simulink model "fir"  (R2019b)
settings: Solver=VariableStepAuto  StartTime=0.0  StopTime=inf  RelTol=1e-3
undefined symbols (not defined in the file): S, vsva2197, xcvc1902, xlfda_numerator
libraries: ModelComposer x2, xbsIndex_r4 x1, dspsrcs4 x1
settings Model: Creator=abehbood  LastModifiedBy=viswanad

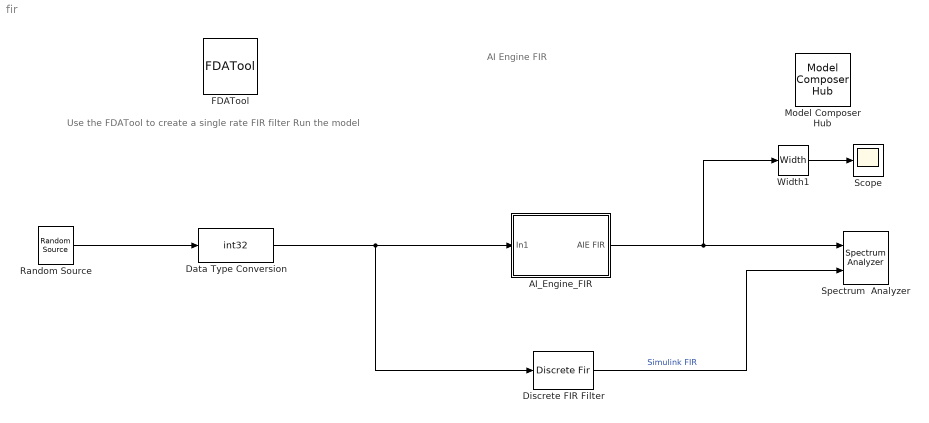
== system fir ==
  note: Use the FDATool to create a single rate FIR filter
      | Run the model
  note: AI Engine FIR
  AI_Engine_FIR : Subsystem
  Data Type Conversion : DataTypeConversion  OutDataTypeStr=int32
  Discrete FIR Filter : DiscreteFir  Coefficients=xlfda_numerator('FDATool')*2^12  InputProcessing=Columns as channels (frame based)  OutDataTypeStr=Inherit: Same as input
  FDATool : xbsIndex_r4/FDATool  block_type=fdatool
      settings: infoedit=FDATool
  Model Composer Hub : ModelComposer/Model Composer Hub  CodeGeneration=off  SubsystemName=AI_Engine_FIR  TargetDirectory=./code  ExportType=AI Engines  IpVendor=xilinx.com  IpLibrary=hls  IpVersion=1.0  IpHWLanguage=Verilog  AieCompilerOptions={}  CreateTestbench=on  TestbenchStackSize=10  RunAieSim=on  AieSimTimeout=50000  LaunchVitisAnalyzer=off  PlotOutput=off  RunX86Sim=off  X86SimTimeout=10  Platform=xilinx_vck190_base_202110_1  ProjDevice=xcvc1902-vsva2197-2MP-e-S  ProjDevicePart=xcvc1902-vsva2197-2MP-e-S  SamplePeriod=-1  ClockFrequency=200  DataPathParallelism=1
  Random Source : dspsrcs4/Random Source  SrcType=Gaussian  NormMethod=Ziggurat  CltLength=12  MinVal=0  MaxVal=1  MeanVal=0  VarVal=50  RepMode=Not repeatable  rawSeed=1  IsInherit=off  SampMode=Discrete  SampTime=1/200e6  SampFrame=256  DataType=Double  OutComplex=Real  OutputFrames=off
  Scope : Scope
  Spectrum  Analyzer : SpectrumAnalyzer  NumInputPorts=2
  Width1 : Width
  wires:
  Discrete FIR Filter/1 -> Spectrum  Analyzer/2  "Simulink FIR"
  Random Source/1 -> Data Type Conversion/1
  Data Type Conversion/1 -> AI_Engine_FIR/1(In1), Discrete FIR Filter/1
  AI_Engine_FIR/1(AIE FIR) -> Width1/1, Spectrum  Analyzer/1
  Width1/1 -> Scope/1

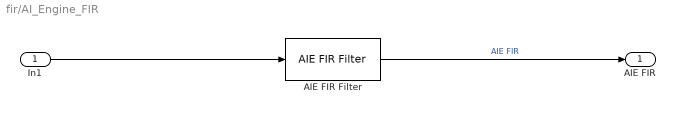
== system fir/AI_Engine_FIR ==
  In1 : Inport
  AIE FIR Filter : ModelComposer/AIE FIR Filter  filter_type=Single Rate  symmetric=off  ipol_factor=1  deci_factor=1  fir_length=length(xlfda_numerator('fir/FDATool'))  coeff=xlfda_numerator('fir/FDATool')*2^12  coef_type=int32  data_type=int32  block_size=256  input_sampling_rate=200  en_casc_length=off  casc_length=4  shift_val=0  rnd_mode=Round to positive infinity
  AIE FIR : Outport
  wires:
  AIE FIR Filter/1 -> AIE FIR/1  "AIE FIR"
  In1/1 -> AIE FIR Filter/1
